simulink model "one_more_example_week9_timedelay"  (R2020b)
settings: Solver=VariableStepAuto  StartTime=0.0  StopTime=10.0  RelTol=1e-6
values from neighbouring files (symbols this model uses):
  kc = 1.57    [one_more_example_timedelay.m]
settings Model: Creator=Douaa  LastModifiedBy=Douaa
settings DataIOCC: ReturnWorkspaceOutputs=off
settings DebuggingCC: AlgebraicLoopMsg=none  ArtificialAlgebraicLoopMsg=none  MultiTaskCondExecSysMsg=none

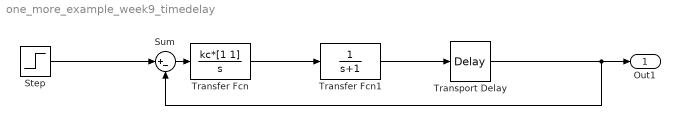
== system one_more_example_week9_timedelay ==
  Step : Step  Time=0  After=1e-6  SampleTime=0
  Sum : Sum  Inputs=|+-
  Transfer Fcn : TransferFcn  Numerator=kc*[1 1]  Denominator=[1 0]
  Transfer Fcn1 : TransferFcn  Denominator=[1 1]
  Transport Delay : TransportDelay
  Out1 : Outport
  wires:
  Step/1 -> Sum/1
  Sum/1 -> Transfer Fcn/1
  Transfer Fcn/1 -> Transfer Fcn1/1
  Transfer Fcn1/1 -> Transport Delay/1
  Transport Delay/1 -> Sum/2, Out1/1
